simulink subsystem "Control_Allocation"  (R2024a)
settings: Solver=VariableStepAuto  StartTime=0.0  StopTime=10.0  RelTol=1e-3
undefined symbols (not defined in the file): FC
settings Model: Creator=gurt1  LastModifiedBy=gurt1
settings RTWCC: GPUComputeCapability=3.5

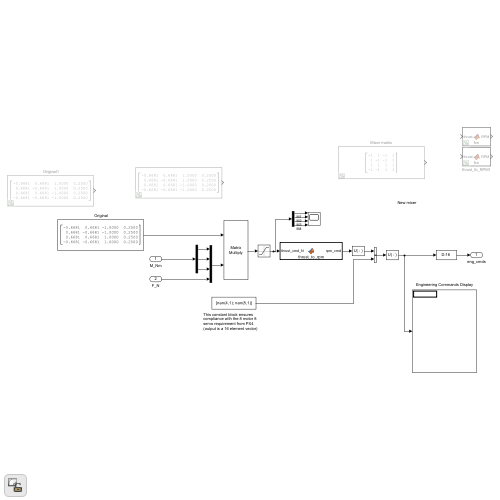
[thumbnail: Simulink's stored preview of the top-level diagram]
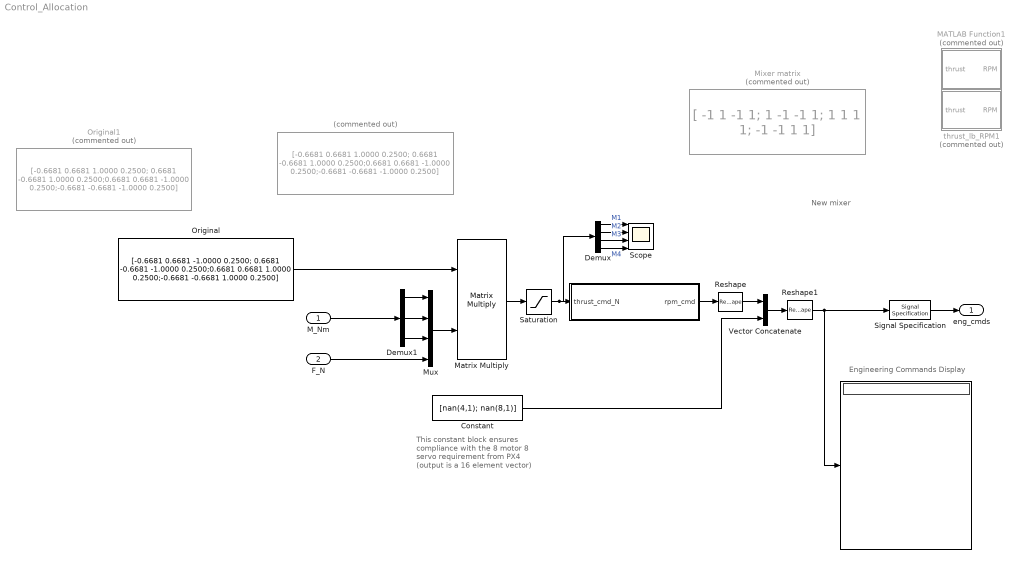
== system Control_Allocation ==
  note: Engineering Commands Display
  note: This constant block ensures compliance with the 8 motor 8 servo requirement from PX4 (output is a 16 element vector)
  note: New mixer
  M_Nm : Inport
  F_N : Inport  Port=2
  " " : Constant  Commented=on  Value=|  OutDataTypeStr=Inherit: Inherit via back propagation  SampleTime=FC.samp_time
      | [-0.6681  0.6681  1.0000  0.2500;
      | 0.6681 -0.6681  1.0000  0.2500;0.6681  0.6681 -1.0000  0.2500;-0.6681 -0.6681 -1.0000  0.2500]
  "   " : MATLAB Function  TreatAsAtomicUnit=on
  "    " : Display
  " Original" : Constant  Value=|  OutDataTypeStr=Inherit: Inherit via back propagation  SampleTime=-1
      | [-0.6681  0.6681  -1.0000  0.2500;
      | 0.6681 -0.6681  -1.0000  0.2500;0.6681  0.6681 1.0000  0.2500;-0.6681 -0.6681 1.0000  0.2500]
  " Original1" : Constant  Commented=on  Value=|  OutDataTypeStr=Inherit: Inherit via back propagation  SampleTime=-1
      | [-0.6681  0.6681  1.0000  0.2500;
      | 0.6681 -0.6681  1.0000  0.2500;0.6681  0.6681 -1.0000  0.2500;-0.6681 -0.6681 -1.0000  0.2500]
  Constant : Constant  Value=[nan(4,1); nan(8,1)]
  Demux : Demux
  Demux1 : Demux  Outputs=3
  MATLAB Function1 : MATLAB Function  Commented=on  TreatAsAtomicUnit=on
  Matrix Multiply : Product  Multiplication=Matrix(*)
  Mixer matrix : Constant  Commented=on  Value="[ -1 1 -1  1; 1  -1 -1  1; 1 1  1  1;  -1  -1  1  1]"  OutDataTypeStr=Inherit: Inherit via back propagation  SampleTime=FC.samp_time
  Mux : Mux
  Reshape : Reshape
  Reshape1 : Reshape
  Saturation : Saturate  UpperLimit=12  LowerLimit=0
  Scope : Scope  NumInputPorts=4
  Signal Specification : SignalSpecification  Dimensions=16
  Vector Concatenate : Concatenate
  thrust_lb_RPM1 : MATLAB Function  Commented=on  TreatAsAtomicUnit=on
  eng_cmds : Outport
  wires:
  Matrix Multiply/1 -> Saturation/1
  Demux/1 -> Scope/1  "M1"
  Demux/2 -> Scope/2  "M2"
  Demux/3 -> Scope/3  "M3"
  Demux/4 -> Scope/4  "M4"
  " Original"/1 -> Matrix Multiply/1
  Vector Concatenate/1 -> Reshape1/1
  Constant/1 -> Vector Concatenate/2
  F_N/1 -> Mux/4
  M_Nm/1 -> Demux1/1
  Demux1/1 -> Mux/1
  Demux1/2 -> Mux/2
  Demux1/3 -> Mux/3
  Mux/1 -> Matrix Multiply/2
  "   "/1(rpm_cmd) -> Reshape/1
  Reshape/1 -> Vector Concatenate/1
  Reshape1/1 -> "    "/1, Signal Specification/1
  Signal Specification/1 -> eng_cmds/1
  Saturation/1 -> "   "/1(thrust_cmd_N), Demux/1

== matlab function Control_Allocation/MATLAB Function1 ==
  data: thrust input; RPM output
function RPM = fcn(thrust)
% Where thrust is in [lb]
RPM = -1064*(thrust.^2)+5752.4*thrust+1660.2;

== matlab function Control_Allocation/thrust_lb_RPM1 ==
  data: thrust input; RPM output
function RPM = fcn(thrust)
% Where thrust is in [lb]
%RPM = -1064*(thrust.^2)+5752.4*thrust+1660.2;

%RPM = -12627.*(thrust.^6)+70491.*(thrust.^5)-152687.*(thrust.^4)+162365.*(thrust.^3)-89894*(thrust.^2)+30170*thrust+440.47;

RPM = -6109.1.*(thrust.^6)+37538.*(thrust.^5)-89942.*(thrust.^4)+106572.*(thrust.^3)-66615*(thrust.^2)+26149*thrust+728.72;

== matlab function Control_Allocation/    ==
  data: thrust_cmd_N input; rpm_cmd output
function rpm_cmd = thrust_to_rpm(thrust_cmd_N)
% Where thrust is in [N]
rpm_cmd = -3.3169.*(thrust_cmd_N.^6) + 67.651.*(thrust_cmd_N.^5) - 532.66.*(thrust_cmd_N.^4) + 2057.2.*(thrust_cmd_N.^3) ...
          - 4192.7.*(thrust_cmd_N.^2) + 5521.9.*thrust_cmd_N + 623.46;
